simulink model "erreurSinus"  (R2016b)
settings: Solver=VariableStepAuto  StartTime=0.0  StopTime=50  RelTol=1e-3  EnableMultiTasking=on
settings Model: Creator=yann  LastModifiedBy=live
settings DataIOCC: LimitDataPoints=on
settings OptimizationCC: LifeSpan=inf
settings DebuggingCC: AllowSymbolicDim=off  SFUnexpectedBacktrackingDiag=warning  SFNoUnconditionalDefaultTransitionDiag=warning  SFExecutionAtInitializationDiag=none
settings ModelReferenceCC: PropagateSignalLabelsOutOfModel=off
settings GRTTargetCC: TargetLangStandard=C89/C90 (ANSI)
settings ConfigComp: CovMetricSettings=dw  CovHtmlReporting=on  CovSaveCumulativeToWorkspaceVar=on  CovSaveSingleToWorkspaceVar=on  CovExternalEMLEnable=off

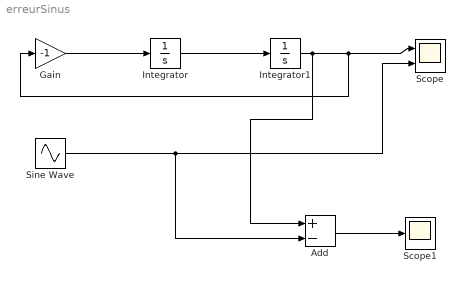
== system erreurSinus ==
  Add : Sum  Inputs=+-
  Gain : Gain  Gain=-1
  Integrator : Integrator  InitialCondition=1
  Integrator1 : Integrator
  Scope : Scope  NumInputPorts=2
  Scope1 : Scope
  Sine Wave : Sin  SampleTime=0
  wires:
  Integrator/1 -> Integrator1/1
  Integrator1/1 -> Add/1, Gain/1, Scope/1
  Gain/1 -> Integrator/1
  Sine Wave/1 -> Add/2, Scope/2
  Add/1 -> Scope1/1
